simulink model "btvn06"  (R2017b)
settings: Solver=ode5  StartTime=0.0  StopTime=60  FixedStep=0.1  RelTol=1e-3
libraries: fuzblock x1
settings Model: Creator=phamt  LastModifiedBy=phamt

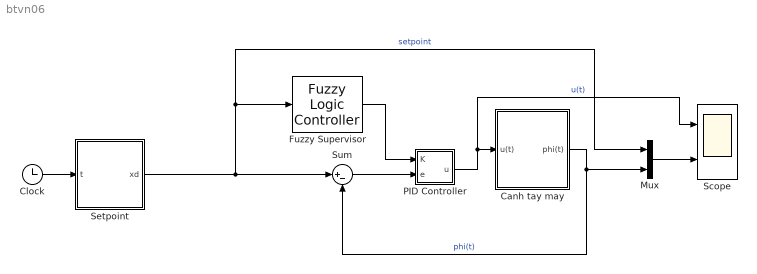
== system btvn06 ==
  Canh tay may : Subsystem  mask{J=0.05, H=1, m=0.1, l=0.4, lc=0.15, B=0.2, g=9.81}
      mask prompts: H "M"
  Clock : Clock
      settings: Decimation=60
  Fuzzy Supervisor : fuzblock/Fuzzy Logic  Controller  FIS='FuzzySugenoPID_SingleTank.fis'  OutputSampleNumber=101  DataType=double  FuzzifiedInputs=off  RuleFiringStrengths=off  RuleOutputs=off  AggregatedOutputs=off  SimulateUsing=Interpreted execution
  Mux : Mux  Inputs=2
  PID Controller : Subsystem  AncestorBlock=simulink_extras/Additional Linear/PID Controller  mask(PID Controller){}
      mask help:
      | Enter expressions for proportional, integral, and derivative terms.
      | P+I/s+Ds
      mask Help: This block implements a PID controller where parameters are entered for the Proportional, Integral and Derivative terms. Unmask this block to see how it works. The derivative term is implemented using a true derivative block.
  Scope : Scope  NumInputPorts=2
  Setpoint : MATLAB Function  TreatAsAtomicUnit=on
  Sum : Sum  Inputs=|+-  SaturateOnIntegerOverflow=on
  wires:
  Fuzzy Supervisor/1 -> PID Controller/1(K)
  Canh tay may/1(phi(t)) -> Sum/2, Mux/2  "phi(t)"
  Mux/1 -> Scope/2
  Sum/1 -> PID Controller/2(e)
  Setpoint/1(xd) -> Sum/1, Fuzzy Supervisor/1, Mux/1  "setpoint"
  Clock/1 -> Setpoint/1(t)
  PID Controller/1(u) -> Scope/1, Canh tay may/1(u(t))  "u(t)"

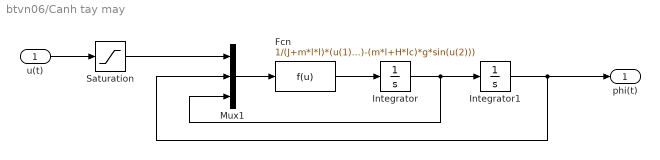
== system btvn06/Canh tay may ==
  u(t) : Inport
  Fcn : Fcn  Expr=1/(J+m*l*l)*(u(1)-B*u(3)-(m*l+H*lc)*g*sin(u(2)))
  Integrator : Integrator  LimitOutput=on  UpperSaturationLimit=pi  LowerSaturationLimit=-10*pi
  Integrator1 : Integrator  LimitOutput=on  UpperSaturationLimit=pi  LowerSaturationLimit=-10*pi
  Mux1 : Mux  Inputs=3
  Saturation : Saturate  UpperLimit=4  LowerLimit=-2
  phi(t) : Outport
  wires:
  Integrator1/1 -> Mux1/2, phi(t)/1
  Mux1/1 -> Fcn/1
  Fcn/1 -> Integrator/1
  Integrator/1 -> Mux1/3, Integrator1/1
  Saturation/1 -> Mux1/1
  u(t)/1 -> Saturation/1

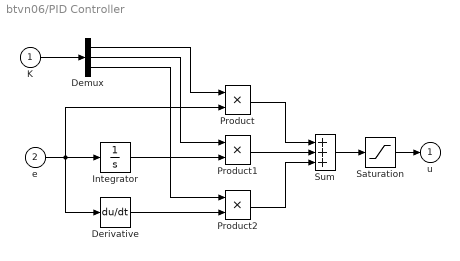
== system btvn06/PID Controller ==
  K : Inport
  e : Inport  Port=2
  Demux : Demux  Outputs=3
  Derivative : Derivative
  Integrator : Integrator
  Product : Product  SaturateOnIntegerOverflow=on  OutDataTypeStr=Inherit: Same as first input
  Product1 : Product  SaturateOnIntegerOverflow=on  OutDataTypeStr=Inherit: Same as first input
  Product2 : Product  SaturateOnIntegerOverflow=on  OutDataTypeStr=Inherit: Same as first input
  Saturation : Saturate  UpperLimit=4  LowerLimit=-2
  Sum : Sum  Inputs=+++  SaturateOnIntegerOverflow=on  InputSameDT=on  OutDataTypeStr=Inherit: Same as first input
  u : Outport  InitialOutput=0
  wires:
  Product/1 -> Sum/1
  e/1 -> Product/2, Integrator/1, Derivative/1
  Sum/1 -> Saturation/1
  K/1 -> Demux/1
  Demux/1 -> Product/1
  Product1/1 -> Sum/2
  Integrator/1 -> Product1/2
  Demux/2 -> Product1/1
  Derivative/1 -> Product2/2
  Product2/1 -> Sum/3
  Demux/3 -> Product2/1
  Saturation/1 -> u/1

== matlab function btvn06/Setpoint ==
  data: t input; xd output
function xd = fcn(t)
if (0<=t) && (t<10)  
    xd = pi/2;
elseif (10<=t) &&(t<20) 
    xd = pi/3;
elseif (20<=t) &&(t<30)  
    xd = pi;
elseif (30<=t) &&(t<40)  
    xd = 2*pi/3;
elseif (40<=t) &&(t<50)  
    xd = pi/6;
elseif (50<=t) &&(t<=60)  
    xd = 3*pi/4;
else xd = 0;
end
end
